simulink model "realtime"  (R2021a)
settings: Solver=ode5  StartTime=0.0  StopTime=500  RelTol=1e-3
undefined symbols (not defined in the file or in its folder): Advantech, PCI
libraries: sldrtlib x4, pid_lib x2, spsLeadLagFilterLib x1
settings Model: SimulationMode=external  Creator=hp  LastModifiedBy=hp
settings SolverCC: AlgebraicLoopSolver=TrustRegion
settings OptimizationCC: EfficientTunableParamExpr=on
settings DebuggingCC: ArithmeticOperatorsInVariantConditions=warning
settings SFSimCC: CustomCodeUndefinedFunction=UseInterfaceOnly  SimTargetLang=C++
settings RTWCC: Description=Simulink Desktop Real-Time (ERT)  SystemTargetFile=sldrtert.tlc  TemplateMakefile=sldrtert.tmf  TargetLang=C++  RTWCompilerOptimization=on
settings CodeAppCC: MaxIdLength=95
settings SimulinkDesktopRealTimeERTCC: TargetFcnLib=ansi_tfl_table_tmw.mat  TargetLibSuffix=_sldrt.lib  TargetPreCompLibLocation=D:\matlab\toolbox\sldrt\lib\win64  GenFloatMathFcnCalls=NOT IN USE  TargetLangStandard=C++03 (ISO)  CodeReplacementLibrary=None  UtilityFuncGeneration=Auto  MultiwordTypeDef=System defined  MultiwordLength=2048  DynamicStringBufferSize=256  GenerateFullHeader=on  InferredTypesCompatibility=off  GenerateSampleERTMain=off  GenerateTestInterfaces=off  ModelReferenceCompliant=on  ParMdlRefBuildCompliant=off  CompOptLevelCompliant=on  ConcurrentExecutionCompliant=off  IncludeMdlTerminateFcn=on  CombineOutputUpdateFcns=off  CombineSignalStateStructs=off  GroupInternalDataByFunction=off  SuppressErrorStatus=off  IncludeFileDelimiter=Auto  ERTCustomFileBanners=off  SupportAbsoluteTime=on  LogVarNameModifier=rt_  MatFileLogging=off  CodeInterfacePackaging=Nonreusable function  PurelyIntegerCode=off  SupportNonFinite=on  SupportComplex=on  SupportContinuousTime=on  SupportNonInlinedSFcns=on  RemoveDisableFunc=off  RemoveResetFunc=off  SupportVariableSizeSignals=on  ParenthesesLevel=Nominal  CastingMode=Nominal  MATLABClassNameForMDSCustomization=Simulink.SoftwareTarget.TargetSpecificTriggerConfigurationBase  ModelStepFunctionPrototypeControlCompliant=off  CPPClassGenCompliant=off  AutosarCompliant=off  MDXCompliant=off  GRTInterface=off  GenerateAllocFcn=off  UseToolchainInfoCompliant=off  GenerateSharedConstants=on  CoderGroups=[]  AccessMethods=[]  LookupTableObjectStructAxisOrder=1,2,3,4,...  LUTObjectStructOrderExplicitValues=Size,Breakpoints,Table  LUTObjectStructOrderEvenSpacing=Size,Breakpoints,Table  ArrayLayout=Column-major  UnsupportedSFcnMsg=error  ERTHeaderFileRootName=$R$E  ERTSourceFileRootName=$R$E  ERTDataFileRootName=$R_data  GenerateASAP2=off  DSAsUniqueAccess=off  InlinedParameterPlacement=Hierarchical  TargetOS=BareBoardExample  MultiInstanceErrorCode=Error  RootIOFormat=Individual arguments  RTWCAPISignals=off  RTWCAPIParams=off  RTWCAPIStates=off  RTWCAPIRootIO=off  ERTSrcFileBannerTemplate=ert_code_template.cgt  ERTHdrFileBannerTemplate=ert_code_template.cgt  ERTDataSrcFileTemplate=ert_code_template.cgt  ERTDataHdrFileTemplate=ert_code_template.cgt  ERTCustomFileTemplate=example_file_process.tlc  EnableDataOwnership=off  SignalDisplayLevel=10  ParamTuneLevel=10  GlobalDataDefinition=Auto  DataDefinitionFile=global.c  GlobalDataReference=Auto  ERTFilePackagingFormat=Modular  RateTransitionBlockCode=Inline  DataReferenceFile=global.h  PreserveExpressionOrder=off  PreserveIfCondition=off  ConvertIfToSwitch=off  PreserveExternInFcnDecls=on  PreserveStaticInFcnDecls=on  SuppressUnreachableDefaultCases=off  EnableSignedLeftShifts=on  EnableSignedRightShifts=on  IndentStyle=K&R  IndentSize=2  NewlineStyle=Default  MaxLineWidth=80  EnableUserReplacementTypes=off  MaxIdInt64=MAX_int64_T  MinIdInt64=MIN_int64_T  MaxIdUint64=MAX_uint64_T  MaxIdInt32=MAX_int32_T  MinIdInt32=MIN_int32_T  MaxIdUint32=MAX_uint32_T  MaxIdInt16=MAX_int16_T  MinIdInt16=MIN_int16_T  MaxIdUint16=MAX_uint16_T  MaxIdInt8=MAX_int8_T  MinIdInt8=MIN_int8_T  MaxIdUint8=MAX_uint8_T  BooleanTrueId=true  BooleanFalseId=false  MemSecPackage=--- None ---  MemSecDataConstants=Default  MemSecDataIO=Default  MemSecDataInternal=Default  MemSecDataParameters=Default  MemSecFuncInitTerm=Default  MemSecFuncExecute=Default  MemSecFuncSharedUtil=Default  GroupConstants=Default  GroupRootInputs=Default  GroupRootOutputs=Default  GroupInternal=Default  GroupParameters=Default  GroupDataTransfer=Default  GroupSharedLocalDataStores=Default  GroupInstanceSpecificParameters=Default  GroupModelData=Default  ArrayContainerType=C-style array  CCListing=off  RebuildAll=off  ExtMode=on  ExtModeTransport=0  ExtModeStaticAlloc=off  ExtModeStaticAllocSize=1000000  ExtModeTesting=off  ExtModeMexFile=sldrtext  ExtModeIntrfLevel=Level1

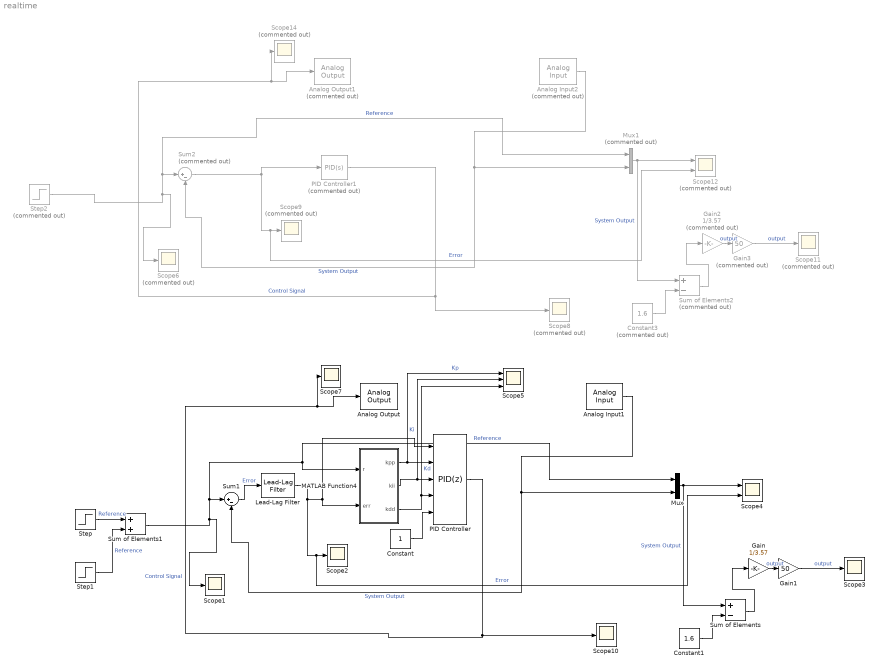
== system realtime ==
  Analog Input1 : sldrtlib/Analog Input  SampleTime=1  MaxMissedTicks=10  ShowMissedTicks=off  YieldWhenWaiting=off  DrvName=Advantech/PCI-1716  DrvAddress=4294967295  DrvOptions=0  Channels=1  RangeMode=1  VoltRange=1  DataType=1
      settings: AttributesFormatString=Advantech\nPCI-1716 [auto]
  Analog Input2 : sldrtlib/Analog Input  Commented=on  SampleTime=1  MaxMissedTicks=10  ShowMissedTicks=off  YieldWhenWaiting=off  DrvName=Advantech/PCI-1716  DrvAddress=4294967295  DrvOptions=0  Channels=1  RangeMode=1  VoltRange=1  DataType=1
      settings: AttributesFormatString=Advantech\nPCI-1716 [auto]
  Analog Output : sldrtlib/Analog Output  SampleTime=1  MaxMissedTicks=10  ShowMissedTicks=off  YieldWhenWaiting=off  DrvName=Advantech/PCI-1716  DrvAddress=4294967295  DrvOptions=0  Channels=1  RangeMode=1  VoltRange=2  InitialValue=0  FinalValue=2.3
      settings: AttributesFormatString=Advantech\nPCI-1716 [auto]
  Analog Output1 : sldrtlib/Analog Output  Commented=on  SampleTime=1  MaxMissedTicks=10  ShowMissedTicks=off  YieldWhenWaiting=off  DrvName=Advantech/PCI-1716  DrvAddress=4294967295  DrvOptions=0  Channels=1  RangeMode=1  VoltRange=2  InitialValue=0  FinalValue=2.3
      settings: AttributesFormatString=Advantech\nPCI-1716 [auto]
  Constant : Constant
  Constant1 : Constant  Value=1.6
  Constant3 : Constant  Commented=on  Value=1.6
  Gain : Gain  Gain=1/3.57
  Gain1 : Gain  Gain=50
  Gain2 : Gain  Commented=on  Gain=1/3.57
  Gain3 : Gain  Commented=on  Gain=50
  Lead-Lag Filter : spsLeadLagFilterLib/Lead-Lag Filter  T1=5e-3  T2=20e-3  Vdc_Init=0  Ts=0
      settings: SourceProductBaseCode=PS
  MATLAB Function4 : MATLAB Function  TreatAsAtomicUnit=on
  Mux : Mux  Inputs=2
  Mux1 : Mux  Commented=on  Inputs=2
  PID Controller : pid_lib/PID Controller  Controller=PID  Form=Parallel  TimeDomain=Discrete-time  UseExternalTs=off  SampleTime=1  IntegratorMethod=Forward Euler  FilterMethod=Forward Euler  ControllerParametersSource=external  P=1  I=1  D=0  UseFilter=on  N=100  TunerSelectOption=Transfer Function Based (PID Tuner App)  InitialConditionSource=internal  InitialConditionForIntegrator=0  InitialConditionForFilter=0  DifferentiatorICPrevScaledInput=0  ExternalReset=none  TrackingMode=off  Kt=1  LimitOutput=on  SatLimitsSource=internal  UpperSaturationLimit=10  LowerSaturationLimit=0  LinearizeAsGain=on  AntiWindupMode=clamping  Kb=1  POutMin=[]  POutMax=[]  IOutMin=[]  IOutMax=[]  DOutMin=[]  DOutMax=[]  NOutMin=[]  NOutMax=[]  SumOutMin=[]  SumOutMax=[]  SaturationOutMin=[]  SaturationOutMax=[]  PParamMin=[]  PParamMax=[]  IParamMin=[]  IParamMax=[]  DParamMin=[]  DParamMax=[]  NParamMin=[]  NParamMax=[]  KbParamMin=[]  KbParamMax=[]  KtParamMin=[]  KtParamMax=[]  KbOutMin=[]  KbOutMax=[]  KtOutMin=[]  KtOutMax=[]  IntegratorOutMin=[]  IntegratorOutMax=[]  FilterOutMin=[]  FilterOutMax=[]  SumI1OutMin=[]  SumI1OutMax=[]  SumI2OutMin=[]  SumI2OutMax=[]  SumI3OutMin=[]  SumI3OutMax=[]  SumI4OutMin=[]  SumI4OutMax=[]  SumDOutMin=[]  SumDOutMax=[]  DifferentiatorOutMin=[]  DifferentiatorOutMax=[]  FilterDiffOutCoefMin=[]  FilterDiffOutCoefMax=[]  ReciprocalOutMin=[]  ReciprocalOutMax=[]  SumDenOutMin=[]  SumDenOutMax=[]  SumNumOutMin=[]  SumNumOutMax=[]  DivideOutMin=[]  DivideOutMax=[]  UdiffTsProdOutMin=[]  UdiffTsProdOutMax=[]  NTsProdOutMin=[]  NTsProdOutMax=[]  UintegralTsProdOutMin=[]  UintegralTsProdOutMax=[]  UngainTsProdOutMin=[]  UngainTsProdOutMax=[]  IntegratorContinuousStateAttributes=''  IntegratorStateMustResolveToSignalObject=off  IntegratorRTWStateStorageClass=Auto  FilterContinuousStateAttributes=''  FilterStateMustResolveToSignalObject=off  FilterRTWStateStorageClass=Auto  ParallelPVariant=ExternalParameters  IdealPVariant=Disabled  IVariant=ExternalParameters  DVariant=ExternalParameters  IntegratorVariant=Discrete  SatVariant=Enabled  AWVariant=DiscClampingParallel  PCopyVariant=Disabled  TRVariant=Disabled  FdbkBlocksVariant=Forward  IdealPFdbkVariant=Disabled  SatFdbkVariant=Disabled  DerivativeFilterVariant=ForwardEulerFilter  NVariant=ExternalParameters  NCopyVariant=Disabled  FilterICVariant=InternalICsFilter  IntegratorICVariant=InternalICs  ExternalResetVariant=Disabled  TRSumVariant=Passthrough  SumFdbkVariant=Disabled  SumVariant=Sum_PID  TsampFilterVariant=InternalTs  TsampNgainVariant=Passthrough  TsampIntegralVariant=Passthrough  ExternalSaturationOutDataTypeStr=Inherit: Same as second input
  PID Controller1 : pid_lib/PID Controller  Commented=on  Controller=PID  Form=Parallel  TimeDomain=Continuous-time  UseExternalTs=off  SampleTime=-1  IntegratorMethod=Forward Euler  FilterMethod=Forward Euler  ControllerParametersSource=internal  P=200  I=3.5  D=0  UseFilter=on  N=1  TunerSelectOption=Transfer Function Based (PID Tuner App)  InitialConditionSource=internal  InitialConditionForIntegrator=0  InitialConditionForFilter=0  DifferentiatorICPrevScaledInput=0  ExternalReset=none  TrackingMode=off  Kt=1  LimitOutput=on  SatLimitsSource=internal  UpperSaturationLimit=10  LowerSaturationLimit=0  LinearizeAsGain=on  AntiWindupMode=clamping  Kb=1  POutMin=[]  POutMax=[]  IOutMin=[]  IOutMax=[]  DOutMin=[]  DOutMax=[]  NOutMin=[]  NOutMax=[]  SumOutMin=[]  SumOutMax=[]  SaturationOutMin=[]  SaturationOutMax=[]  PParamMin=[]  PParamMax=[]  IParamMin=[]  IParamMax=[]  DParamMin=[]  DParamMax=[]  NParamMin=[]  NParamMax=[]  KbParamMin=[]  KbParamMax=[]  KtParamMin=[]  KtParamMax=[]  KbOutMin=[]  KbOutMax=[]  KtOutMin=[]  KtOutMax=[]  IntegratorOutMin=[]  IntegratorOutMax=[]  FilterOutMin=[]  FilterOutMax=[]  SumI1OutMin=[]  SumI1OutMax=[]  SumI2OutMin=[]  SumI2OutMax=[]  SumI3OutMin=[]  SumI3OutMax=[]  SumI4OutMin=[]  SumI4OutMax=[]  SumDOutMin=[]  SumDOutMax=[]  DifferentiatorOutMin=[]  DifferentiatorOutMax=[]  FilterDiffOutCoefMin=[]  FilterDiffOutCoefMax=[]  ReciprocalOutMin=[]  ReciprocalOutMax=[]  SumDenOutMin=[]  SumDenOutMax=[]  SumNumOutMin=[]  SumNumOutMax=[]  DivideOutMin=[]  DivideOutMax=[]  UdiffTsProdOutMin=[]  UdiffTsProdOutMax=[]  NTsProdOutMin=[]  NTsProdOutMax=[]  UintegralTsProdOutMin=[]  UintegralTsProdOutMax=[]  UngainTsProdOutMin=[]  UngainTsProdOutMax=[]  IntegratorContinuousStateAttributes=''  IntegratorStateMustResolveToSignalObject=off  IntegratorRTWStateStorageClass=Auto  FilterContinuousStateAttributes=''  FilterStateMustResolveToSignalObject=off  FilterRTWStateStorageClass=Auto  ParallelPVariant=InternalParameters  IdealPVariant=Disabled  IVariant=InternalParameters  DVariant=InternalParameters  IntegratorVariant=Continuous  SatVariant=Enabled  AWVariant=ContClampingParallel  PCopyVariant=Disabled  TRVariant=Disabled  FdbkBlocksVariant=Forward  IdealPFdbkVariant=Disabled  SatFdbkVariant=Disabled  DerivativeFilterVariant=ContFilter  NVariant=InternalParameters  NCopyVariant=Disabled  FilterICVariant=InternalICsFilter  IntegratorICVariant=InternalICs  ExternalResetVariant=Disabled  TRSumVariant=Passthrough  SumFdbkVariant=Disabled  SumVariant=Sum_PID  TsampFilterVariant=InternalTs  TsampNgainVariant=Passthrough  TsampIntegralVariant=Passthrough  ExternalSaturationOutDataTypeStr=Inherit: Same as second input
  Scope{1..3,7,10} (5 alike) : Scope
  Scope{6,8..9,11,14} (5 alike) : Scope  Commented=on
  Scope12 : Scope  Commented=on  NumInputPorts=2
  Scope4 : Scope  NumInputPorts=2
  Scope5 : Scope  NumInputPorts=3
  Step : Step  Time=0  Before=3.5  After=3.5  SampleTime=1
  Step1 : Step  Time=350  SampleTime=1
  Step2 : Step  Commented=on  Time=0  Before=3.5  After=3.5  SampleTime=1
  Sum of Elements : Sum  Inputs=+-
  Sum of Elements1 : Sum
  Sum of Elements2 : Sum  Commented=on  Inputs=+-
  Sum1 : Sum  Inputs=|+-  SaturateOnIntegerOverflow=on
  Sum2 : Sum  Commented=on  Inputs=|+-  SaturateOnIntegerOverflow=on
  wires:
  Lead-Lag Filter/1 -> Scope4/2, Scope2/1, MATLAB Function4/2(err), PID Controller/1  "Error"
  PID Controller/1 -> Scope7/1, Analog Output/1, Scope10/1  "Control Signal"
  MATLAB Function4/3(kdd) -> Scope5/3, PID Controller/4  "Kd"
  MATLAB Function4/2(kii) -> Scope5/2, PID Controller/3  "Ki"
  MATLAB Function4/1(kpp) -> Scope5/1, PID Controller/2  "Kp"
  Mux/1 -> Scope4/1, Sum of Elements/1  "System Output"
  Sum of Elements1/1 -> Scope1/1, Mux/1, MATLAB Function4/1(r), Sum1/1  "Reference"
  Analog Input1/1 -> Sum1/2, Mux/2  "System Output"
  Constant/1 -> PID Controller/5
  Constant1/1 -> Sum of Elements/2
  Sum of Elements/1 -> Gain/1
  Gain/1 -> Gain1/1  "output"
  Gain1/1 -> Scope3/1  "output"
  Step/1 -> Sum of Elements1/1  "Reference"
  Step1/1 -> Sum of Elements1/2  "Reference"
  Sum of Elements2/1 -> Gain2/1
  Step2/1 -> Scope6/1, Mux1/1, Sum2/1  "Reference"
  Gain2/1 -> Gain3/1  "output"
  PID Controller1/1 -> Scope8/1, Scope14/1, Analog Output1/1  "Control Signal"
  Analog Input2/1 -> Sum2/2, Mux1/2  "System Output"
  Sum2/1 -> PID Controller1/1, Scope12/2, Scope9/1  "Error"
  Gain3/1 -> Scope11/1  "output"
  Constant3/1 -> Sum of Elements2/2
  Mux1/1 -> Scope12/1, Sum of Elements2/1  "System Output"
  Sum1/1 -> Lead-Lag Filter/1  "Error"

== matlab function realtime/MATLAB Function4 ==
  settings: updateMethod=DISCRETE  sampleTime=1
  data: r input; err input; kpp output; kii output; kdd output
function [kpp,kii,kdd]  = fcn(r,err)
persistent Wij_c_p W1j_c_p S_prev_c_p e_prev_c_p u_prev_c_p u_prev_e_P control_prev
        if isempty(Wij_c_p)
        Wij_c_p = 0.05*rand(4,4);
        end
        if isempty(W1j_c_p)
        W1j_c_p = 0.05*rand(1,4);
        end
        if isempty(S_prev_c_p)
        S_prev_c_p = [0.1 0.2 0.3 0.4];
        end
        if isempty(e_prev_c_p)
        e_prev_c_p = 1;
        end
        if isempty(err)
        err = 1;
        end
        if isempty(u_prev_c_p)
        u_prev_c_p = 0;
        end
        if isempty(u_prev_e_P)
        u_prev_e_P = 0.05;
        end
        if isempty(control_prev)
        control_prev = 0;
        end
       % ********
           persistent e e_prev1 e_prev2 e_prev3 error_status
       error_status = 1;
       while true
            if isempty(e)
                e = err
                e_prev1 = 1
                e_prev2 = 1
                e_prev3 = 1
                error_status = 2;
                break
            elseif error_status == 2
                e_prev1 = e
                e = err
                e_prev2
                e_prev3
                error_status = 3
                break
            elseif error_status == 3
                e_prev2 = e_prev1
                e_prev1  = e
                e = err
                e_prev3
                error_status == 4
                break
            elseif error_status == 4
                e_prev3 =e_prev2
                e_prev2 = e_prev1
                e_prev1 = e
                e = err
                error_status == 5
                break
            else
                e_prev3 =e_prev2
                e_prev2 = e_prev1
                e_prev1 = e
                e = err
                break
            end
       end
       %***********
       persistent xp xp_prev1 xp_prev2 xp_prev3 xp_status
       xp_status = 1;
       while true
            if isempty(xp)
                xp = r
                xp_prev1 = 1
                xp_prev2 = 1
                xp_prev3 = 1
                xp_status = 2;
                break
            elseif xp_status == 2
                xp_prev1 = xp
                xp = r
                xp_prev2
                xp_prev3
                xp_status = 3
                break
            elseif xp_status == 3
                xp_prev2 = xp_prev1
                xp_prev1  = xp
                xp = r
                xp_prev3
                xp_status == 4
                break
            elseif xp_status == 4
                xp_prev3 =xp_prev2
                xp_prev2 = xp_prev1
                xp_prev1 = xp
                xp = r
                xp_status == 5
                break
            else
                xp_prev3 =xp_prev2
                xp_prev2 = xp_prev1
                xp_prev1 = xp
                xp = r
                break
            end
       end
       %******
       persistent Kp Ki Kd Kp_prev Ki_prev Kd_prev
        if isempty(Kp)
        Kp = 200;
        end
        if isempty(Ki)
        Ki = 3.5;
        end
        if isempty(Kd)
        Kd = 0.0043;
        end
        if isempty(Kp_prev)
        Kp_prev = 0;
        end
        if isempty(Ki_prev)
        Ki_prev = 0;
        end
        if isempty(Kd_prev)
        Kd_prev = 0;
        end

% input layer
net1_c_p = [xp;xp_prev1;xp_prev2;xp_prev3];
O1_c_p = net1_c_p;

% hidden layyer 
S_c_p = zeros (1,4);
 for j = 1:4
       S_c_p(j) = tanh(Wij_c_p(j,1)*xp+Wij_c_p(j,2)*xp_prev1 + Wij_c_p(j,3)*xp_prev2 + Wij_c_p(j,4)*xp_prev3);
 end
O2_c_p = zeros(1,4);
O2_c_p = [S_c_p(1),S_c_p(2),S_c_p(3),S_c_p(4)];

%output layer
net3_c_p = 0;
net3_c_p = W1j_c_p.*O2_c_p;
u_c_p = 0.5*(1+tanh(net3_c_p(1,1)+ net3_c_p(1,2) + net3_c_p(1,3)+net3_c_p(1,4)));

%% updating weights
B_c_p = 0.025;
d_c_p = u_prev_e_P;
sigma_c_p = sqrt(B_c_p)*e_prev1 + d_c_p;

%W1j updating
for j = 1 :4
    W1j_c_p(j) = sigma_c_p/(4*(S_prev_c_p(j))); 
end

%Wij updating
for j = 1:4
    Wij_c_p(j,1) = (1/(4*xp))*atanh(sigma_c_p/(4*W1j_c_p(1,j))); 
end
for j = 1:4
    Wij_c_p(j,2) = (1/(4*xp_prev1))*atanh(sigma_c_p/(4*W1j_c_p(1,j))); 
end
for j = 1:4
    Wij_c_p(j,3) = (1/(4*xp_prev2))*atanh(sigma_c_p/(4*W1j_c_p(1,j))); 
end
for j = 1:4
    Wij_c_p(j,4) = (1/(4*xp_prev3))*atanh(sigma_c_p/(4*W1j_c_p(1,j))); 
end

%% NNE
persistent Wij_e_p W1j_e_p S_prev_e_p e_prev_e_p  
        if isempty(Wij_e_p)
        Wij_e_p = 0.05*rand(4,4);
        end
        if isempty(W1j_e_p)
        W1j_e_p = 0.05*rand(1,4);
        end
        if isempty(S_prev_e_p)
        S_prev_e_p = [0.1 0.2 0.3 0.4];
        end
        if isempty(e_prev_e_p)
        e_prev_e_p = 1;
        end
    
% input layer
net1_e_p = [xp;xp_prev1;xp_prev2;xp_prev3];
O1_e_p = net1_e_p;

% hidden layyer 
S_e_p = zeros (1,4);
 for j = 1:4
       S_e_p(j) = tanh(Wij_e_p(j,1)*xp+Wij_e_p(j,2)*xp_prev1 + Wij_e_p(j,3)*xp_prev2 + Wij_e_p(j,4)*xp_prev3);
 end
O2_e_p = zeros(1,4);
O2_e_p = [S_e_p(1),S_e_p(2),S_e_p(3),S_e_p(4)];

%output layer
net3_e_p = 0;
net3_e_p = W1j_e_p.*O2_e_p;
u_e_p = 0.5*(1+tanh(net3_e_p(1,1)+ net3_e_p(1,2) + net3_e_p(1,3)+net3_e_p(1,4)));

%% updating weights
e_e_p = u_e_p - u_c_p;
B_e_p = 0.025;
d_e_p = u_c_p;
u_c_p = u_c_p*80/3.33;
sigma_e_p = sqrt(B_e_p)*e_prev_e_p + d_e_p;
for j = 1 :4
    W1j_e_p(j) = sigma_e_p/(4*(S_prev_e_p(j)));
end

for j = 1:4
    Wij_e_p(j,1) = (1/(4*xp))*atanh(sigma_e_p/(4*W1j_e_p(1,j))); 
end
for j = 1:4
    Wij_e_p(j,2) = (1/(4*xp_prev1))*atanh(sigma_e_p/(4*W1j_e_p(1,j))); 
end
for j = 1:4
    Wij_e_p(j,3) = (1/(4*xp_prev2))*atanh(sigma_e_p/(4*W1j_e_p(1,j))); 
end
for j = 1:4
    Wij_e_p(j,4) = (1/(4*xp_prev3))*atanh(sigma_e_p/(4*W1j_e_p(1,j))); 
end

%**************
S_prev_c_p = S_c_p;
e_prev_c_p = err;
S_prev_e_p = S_e_p;
e_prev_e_p = e_e_p;
u_prev_e_P = u_e_p;

%% NNI
persistent Wij_c_i W1j_c_i S_prev_c_i e_prev_c_i u_prev_c_i u_prev_e_i error_integral
    if isempty(Wij_c_i)
        Wij_c_i = 0.05*rand(4,4);
    end
    if isempty(W1j_c_i)
        W1j_c_i = 0.05*rand(1,4);
    end
        if isempty(S_prev_c_i)
        S_prev_c_i = [0.1 0.2 0.3 0.4];
        end
        if isempty(e_prev_c_i)
        e_prev_c_i = 1;
        end
        if isempty(err)
        err = 1;
        end
        if isempty(u_prev_c_i)
        u_prev_c_i = 0;
        end
        if isempty(u_prev_e_i)
        u_prev_e_i = 0.05;
        end
        if isempty(error_integral)
        error_integral = 1;
        end

    
% input layer
net1_c_i = [xp;xp_prev1;xp_prev2;xp_prev3];
O1_c_i = net1_c_i;

% hidden layyer 
S_c_i = zeros (1,4);
 for j = 1:4
       S_c_i(j) = tanh(Wij_c_i(j,1)*xp+Wij_c_i(j,2)*xp_prev1 + Wij_c_i(j,3)*xp_prev2 + Wij_c_i(j,4)*xp_prev3);
 end
O2_c_i = zeros(1,4);
O2_c_i = [S_c_i(1),S_c_i(2),S_c_i(3),S_c_i(4)]; 
%output layer
net3_c_i = 0;
net3_c_i = W1j_c_i.*O2_c_i;
u_c_i = 0.5*(1+tanh(net3_c_i(1,1)+ net3_c_i(1,2) + net3_c_i(1,3)+net3_c_i(1,4)));

%% updating weights
B_c_i = 0.025;
d_c_i = u_prev_e_i;
sigma_c_i = sqrt(B_c_i)*error_integral + d_c_i;
error_integral = e + error_integral;
for j = 1 :4
    W1j_c_i(j) = sigma_c_i/(4*(S_prev_c_i(j))); 
end

for j = 1:4
    Wij_c_i(j,1) = (1/(4*xp))*atanh(sigma_c_i/(4*W1j_c_i(1,j)));
end
for j = 1:4
    Wij_c_i(j,2) = (1/(4*xp_prev1))*atanh(sigma_c_i/(4*W1j_c_i(1,j))); 
end
for j = 1:4
    Wij_c_i(j,3) = (1/(4*xp_prev2))*atanh(sigma_c_i/(4*W1j_c_i(1,j))); 
end
for j = 1:4
    Wij_c_i(j,4) = (1/(4*xp_prev3))*atanh(sigma_c_i/(4*W1j_c_i(1,j))); 
end

%% NNE
persistent Wij_e_i W1j_e_i S_prev_e_i e_prev_e_i  
    if isempty(Wij_e_i)
        Wij_e_i = 0.05*rand(4,4);
    end
    if isempty(W1j_e_i)
        W1j_e_i = 0.05*rand(1,4);
    end
        if isempty(S_prev_e_i)
        S_prev_e_i = [0.1 0.2 0.3 0.4];
        end
        if isempty(e_prev_e_i)
        e_prev_e_i = 1;
        end
    
% input layer
net1_e_i = [xp;xp_prev1;xp_prev2;xp_prev3];
O1_e_i = net1_e_i;
% hidden layyer 
S_e_i = zeros (1,4);
 for j = 1:4
       S_e_i(j) = tanh(Wij_e_i(j,1)*xp+Wij_e_i(j,2)*xp_prev1 + Wij_e_i(j,3)*xp_prev2 + Wij_e_i(j,4)*xp_prev3);
 end
O2_e_i = zeros(1,4);
O2_e_i = [S_e_i(1),S_e_i(2),S_e_i(3),S_e_i(4)]; 
%output layer
net3_e_i = 0;
net3_e_i = W1j_e_i.*O2_e_i;
u_e_i = 0.5*(1+tanh(net3_e_i(1,1)+ net3_e_i(1,2) + net3_e_i(1,3)+net3_e_i(1,4)));

%% updating weights
e_e_i = u_e_i - u_c_i;
B_e_i = 0.025;
d_e_i = u_c_i;
u_c_i = u_c_i*0.7;
sigma_e_i = sqrt(B_e_i)*e_prev_e_i + d_e_i;
for j = 1 :4
    W1j_e_i(j) = sigma_e_i/(4*(S_prev_e_i(j))); 
end

for j = 1:4
    Wij_e_i(j,1) = (1/(4*xp))*atanh(sigma_e_i/(4*W1j_e_i(1,j))); 
end
for j = 1:4
    Wij_e_i(j,2) = (1/(4*xp_prev1))*atanh(sigma_e_i/(4*W1j_e_i(1,j))); 
end
for j = 1:4
    Wij_e_i(j,3) = (1/(4*xp_prev2))*atanh(sigma_e_i/(4*W1j_e_i(1,j))); 
end
for j = 1:4
    Wij_e_i(j,4) = (1/(4*xp_prev3))*atanh(sigma_e_i/(4*W1j_e_i(1,j))); 
end

%**************
S_prev_c_i = S_c_i;
e_prev_c_i = err;
S_prev_e_i = S_e_i;
e_prev_e_i = e_e_i;
u_prev_e_i = u_e_i;

%% NND
persistent Wij_c_d W1j_c_d S_prev_c_d e_prev_c_d u_prev_c_d u_prev_e_d error_derivative
    if isempty(Wij_c_d)
        Wij_c_d = 0.05*rand(4,4);
    end
    if isempty(W1j_c_d)
        W1j_c_d = 0.05*rand(1,4);
    end
        if isempty(S_prev_c_d)
        S_prev_c_d = [0.1 0.2 0.3 0.4];
        end
        if isempty(e_prev_c_d)
        e_prev_c_d = 1;
        end
        if isempty(u_prev_c_d)
        u_prev_c_d = 0;
        end
        if isempty(u_prev_e_d)
        u_prev_e_d = 0.05;
        end
        if isempty(error_derivative)
        error_derivative = 1;
        end

   
% input layer
net1_c_d = [xp;xp_prev1;xp_prev2;xp_prev3];
O1_c_d = net1_c_d;
% hidden layyer 
S_c_d = zeros (1,4);
 for j = 1:4
       S_c_d(j) = tanh(Wij_c_d(j,1)*xp+Wij_c_d(j,2)*xp_prev1 + Wij_c_d(j,3)*xp_prev2 + Wij_c_d(j,4)*xp_prev3);
 end

O2_c_d = zeros(1,4);
O2_c_d = [S_c_d(1),S_c_d(2),S_c_d(3),S_c_d(4)]; 
%output layer
net3_c_d = 0;
net3_c_d = W1j_c_d.*O2_c_d;
u_c_d = 0.5*(1+tanh(net3_c_d(1,1)+ net3_c_d(1,2) + net3_c_d(1,3)+net3_c_d(1,4)));

%% updating weights
B_c_d = 0.025;
d_c_d = u_prev_e_d;

sigma_c_d = sqrt(B_c_d)*error_derivative + d_c_d;
 error_derivative = (e - e_prev1)/0.002; 
for j = 1 :4
    W1j_c_d(j) = sigma_c_d/(4*(S_prev_c_d(j))); 
end
% W1j = sigma / (4*S_prev);

for j = 1:4
    Wij_c_d(j,1) = (1/(4*xp))*atanh(sigma_c_d/(4*W1j_c_d(1,j))); 
end
for j = 1:4
    Wij_c_d(j,2) = (1/(4*xp_prev1))*atanh(sigma_c_d/(4*W1j_c_d(1,j))); 
end
for j = 1:4
    Wij_c_d(j,3) = (1/(4*xp_prev2))*atanh(sigma_c_d/(4*W1j_c_d(1,j))); 
end
for j = 1:4
    Wij_c_d(j,4) = (1/(4*xp_prev3))*atanh(sigma_c_d/(4*W1j_c_d(1,j))); 
end
%% NNE
persistent Wij_e_d W1j_e_d S_prev_e_d e_prev_e_d  
    if isempty(Wij_e_d)
        Wij_e_d = 0.05*rand(4,4);
    end
    if isempty(W1j_e_d)
        W1j_e_d = 0.05*rand(1,4);
    end
        if isempty(S_prev_e_d)
        S_prev_e_d = [0.1 0.2 0.3 0.4];
        end
        if isempty(e_prev_e_d)
        e_prev_e_d = 1;
        end
    
% input layer
net1_e_d = [xp;xp_prev1;xp_prev2;xp_prev3];
O1_e_d = net1_e_d;
% hidden layyer 
S_e_d = zeros (1,4);
 for j = 1:4
       S_e_d(j) = tanh(Wij_e_d(j,1)*xp+Wij_e_d(j,2)*xp_prev1 + Wij_e_d(j,3)*xp_prev2 + Wij_e_d(j,4)*xp_prev3);
 end
O2_e_d = zeros(1,4);
O2_e_d = [S_e_d(1),S_e_d(2),S_e_d(3),S_e_d(4)]; 
%output layer
net3_e_d = 0;
net3_e_d = W1j_e_d.*O2_e_d;
u_e_d = 0.5*(1+tanh(net3_e_d(1,1)+ net3_e_d(1,2) + net3_e_d(1,3)+net3_e_d(1,4)));
%% updating weights
e_e_d = u_e_d - u_c_d;
B_e_d = 0.8;
d_e_d = u_c_d;
u_c_d = u_c_d*0.001;
sigma_e_d = sqrt(B_e_d)*e_prev_e_d + d_e_d;
for j = 1 :4
    W1j_e_d(j) = sigma_e_d/(4*(S_prev_e_d(j)));
end

for j = 1:4
    Wij_e_d(j,1) = (1/(4*xp))*atanh(sigma_e_d/(4*W1j_e_d(1,j))); 
end
for j = 1:4
    Wij_e_d(j,2) = (1/(4*xp_prev1))*atanh(sigma_e_d/(4*W1j_e_d(1,j))); 
end
for j = 1:4
    Wij_e_d(j,3) = (1/(4*xp_prev2))*atanh(sigma_e_d/(4*W1j_e_d(1,j))); 
end
for j = 1:4
    Wij_e_d(j,4) = (1/(4*xp_prev3))*atanh(sigma_e_d/(4*W1j_e_d(1,j))); 
end


Kp = u_c_p;
Ki = u_c_i;
Kd = u_c_d;
Kp_prev = Kp;
Ki_prev = Ki;
Kd_prev = Kd;
kpp =Kp;
kii=Ki;
kdd=Kd;

%**************
S_prev_c_d = S_c_d;
e_prev_c_d = err;
S_prev_e_d = S_e_d;
e_prev_e_d = e_e_d;
u_prev_e_d = u_e_d;
